simulink model "Aufgabe_10_2_2_Arbeitsband"  (R2023a)
settings: Solver=VariableStepAuto  StartTime=0.0  StopTime=10.0  RelTol=1e-3
settings Model: Creator=Junle  LastModifiedBy=ASUS
settings RTWCC: GPUComputeCapability=5.0

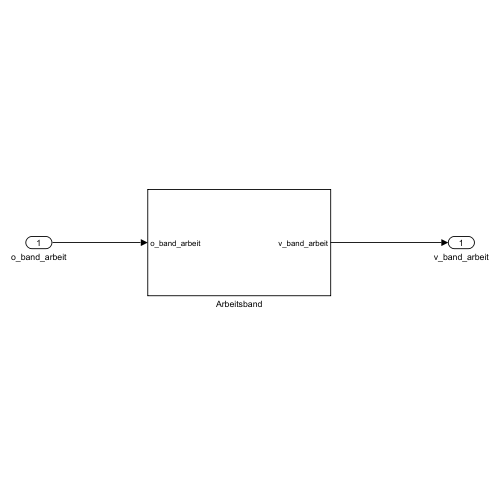
[thumbnail: Simulink's stored preview of the top-level diagram]
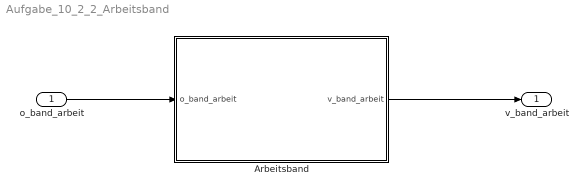
== system Aufgabe_10_2_2_Arbeitsband ==
  o_band_arbeit : Inport
  Arbeitsband : Subsystem
  v_band_arbeit : Outport
  wires:
  o_band_arbeit/1 -> Arbeitsband/1(o_band_arbeit)
  Arbeitsband/1(v_band_arbeit) -> v_band_arbeit/1

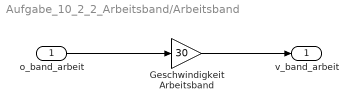
== system Aufgabe_10_2_2_Arbeitsband/Arbeitsband ==
  o_band_arbeit : Inport
  Geschwindigkeit Arbeitsband : Gain  Gain=30
  v_band_arbeit : Outport
  wires:
  Geschwindigkeit Arbeitsband/1 -> v_band_arbeit/1
  o_band_arbeit/1 -> Geschwindigkeit Arbeitsband/1
